simulink model "debug_BoschIMU"  (Simulink 9.0)
settings: Solver=FixedStepDiscrete  StartTime=0.0  StopTime=inf  FixedStep=0.01  RelTol=1e-3  EnableMultiTasking=on
InitFcn:
  | ROBOT_DOF=23;
libraries: WBToolboxLibrary x2
settings Model: SuppressorTable=22 serialization::archive 11 0 6 0 0 0 1 0  Creator=DanielePucci  LastModifiedBy=gnava
settings DataIOCC: LimitDataPoints=on  SaveFormat=Dataset
settings DebuggingCC: UnderspecifiedInitializationDetection=Simplified  MergeDetectMultiDrivingBlocksExec=error  AllowSymbolicDim=off
settings HardwareCC: ProdBitPerPointer=64  ProdBitPerSizeT=64  ProdBitPerPtrDiffT=64  ProdLargestAtomicFloat=Float  ProdIntDivRoundTo=Zero  ProdEndianess=LittleEndian  ProdWordSize=64  ProdHWDeviceType=Intel->x86-64 (Windows64)

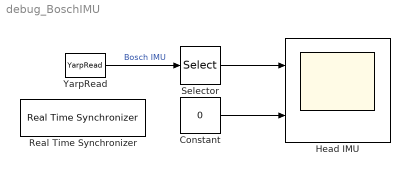
== system debug_BoschIMU ==
  Constant : Constant  Value=0
  Head IMU : Scope  NumInputPorts=2
  Real Time Synchronizer : WBToolboxLibrary/Utilities/Real Time Synchronizer  period=0.01
      settings: SourceProductName=WholeBodyToolbox
  Selector : Selector  InputPortWidth=12  IndexOptions=Index vector (dialog)  Indices=[4:6]  OutputSizes=1
  YarpRead : WBToolboxLibrary/Utilities/YarpRead  portName='/icub/inertial'  signalSize=12  timeout=0.5  blocking=off  timestamp=off  autoconnect=on  errorOnConnection=off
      settings: SourceProductName=WholeBodyToolbox
  wires:
  YarpRead/1 -> Selector/1  "Bosch IMU"
  Selector/1 -> Head IMU/1
  Constant/1 -> Head IMU/2
